simulink model "sldemo2_househeat"  (R2020b)
settings: Solver=ode45  StartTime=0.0  StopTime=48  FixedStep=1  RelTol=1e-3  AbsTol=1e-6
model workspace (MATLAB code in the model file):
  | % load initial conditions and physical properties from file
  | 
  | sldemo_househeat_data
values from neighbouring files (symbols this model uses):
  c = 1005.4    [sldemo_househeat_data.m]
  cost = 0.09/3.6e6    (= 2.5e-08)    [sldemo_househeat_data.m]
  M = (lenHouse*widHouse*htHouse+tan(pitRoof)*widHouse*lenHouse)*densAir    [sldemo_househeat_data.m]
  Mdot = 3600    [sldemo_househeat_data.m]
  Req = RWall*RWindow/(RWall + RWindow)    [sldemo_househeat_data.m]
  TCooler = 5    [sldemo_househeat_data.m]
  THeater = 50    [sldemo_househeat_data.m]
  TinIC = 20    [sldemo_househeat_data.m]
libraries: simulink_extras x3
Description:
  | Thermal Model of a House
  | 
  | This demo illustrates how you can use Simulink(R) to create the thermal model of
  | a house. This system models the outdoor environment, the thermal
  | characteristics of the house, and the house heating system.
  | 
  | The sldemo_househeat_data.m file initializes data in the model workspace.
  | To make changes, you can edit the model workspace directly or edit the MATLAB(R) file
  | and re-load the model workspace.
  | 
  | To view the model workspace, select View > Model Explorer
  | from the Simulink editor.
  | 
  | Note: Time is given in units of hours
settings Model: ExtModeTrigMode=oneshot  ExtModeArmWhenConnect=off  ExtModeAutoUpdateStatusClock=off  Creator=The MathWorks, Inc.  LastModifiedBy=91998
settings SolverCC: AutoScaleAbsTol=off
settings DataIOCC: ExternalInput=[]  InitialState=[]  SaveFormat=Array  SaveOutput=off  SaveTime=off  SignalLoggingName=sldemo_househeat_output
settings OptimizationCC: BlockReduction=off  BooleanDataType=off  ExpressionDepthLimit=2147483647  InitFltsAndDblsToZero=on  LifeSpan=inf  BufferReusableBoundary=off
settings DebuggingCC: SaveWithParameterizedLinksMsg=none  UnderspecifiedInitializationDetection=Classic  MergeDetectMultiDrivingBlocksExec=none  SignalResolutionControl=TryResolveAllWithWarning  MultiTaskDSMMsg=warning  MultiTaskCondExecSysMsg=none  IntegerOverflowMsg=none  FcnCallInpInsideContextMsg=warning  BusObjectLabelMismatch=none  StateNameClashWarn=warning  SFUnexpectedBacktrackingDiag=warning  SFNoUnconditionalDefaultTransitionDiag=warning  SFExecutionAtInitializationDiag=none  IntegerSaturationMsg=none  ArithmeticOperatorsInVariantConditions=warning
settings HardwareCC: ProdBitPerPointer=32  ProdBitPerSizeT=32  ProdBitPerPtrDiffT=32  ProdLargestAtomicFloat=None  ProdIntDivRoundTo=Undefined  ProdEndianess=Unspecified  ProdWordSize=32  ProdHWDeviceType=32-bit Generic  TargetUnknown=on
settings ModelReferenceCC: PropagateSignalLabelsOutOfModel=off
settings SFSimCC: SimUseLocalCustomCode=off  CustomCodeUndefinedFunction=UseInterfaceOnly
settings RTWCC: RTWUseLocalCustomCode=off
settings CodeAppCC: StateflowObjectComments=on
settings GRTTargetCC: TargetFcnLib=ansi_tfl_tmw.mat  TargetLangStandard=C89/C90 (ANSI)  CombineOutputUpdateFcns=off  GRTInterface=on
settings ConfigComp: CovMetricSettings=dw  CovSaveCumulativeToWorkspaceVar=on  CovSaveSingleToWorkspaceVar=on  CovExternalEMLEnable=off

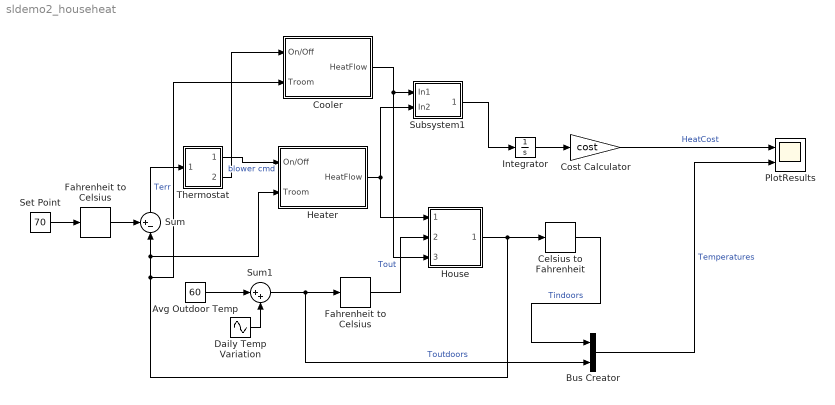
== system sldemo2_househeat ==
  Avg Outdoor Temp : Constant  Value=60
  Bus Creator : BusCreator  Inputs=3
  Celsius to Fahrenheit : simulink_extras/Transformations/Celsius to Fahrenheit
      settings: SourceProductBaseCode=SL
  Cooler : Subsystem
  Cost Calculator : Gain  Gain=cost  SaturateOnIntegerOverflow=on  OutDataTypeStr=Inherit: Same as input  ParamDataTypeStr=Inherit: Same as input
  Daily Temp Variation : Sin  Amplitude=30  Frequency=2*pi/24  SampleTime=0
  Fahrenheit to Celsius : simulink_extras/Transformations/Fahrenheit to Celsius
      settings: SourceProductBaseCode=SL
  "Fahrenheit to Celsius " : simulink_extras/Transformations/Fahrenheit to Celsius
      settings: SourceProductBaseCode=SL
  Heater : Subsystem
  House : Subsystem
      mask Display: image(fullfile(matlabroot,'toolbox','simulink','simdemos','simgeneral','images','HouseHeatHousePix.svg'))
  Integrator : Integrator
  PlotResults : Scope  NumInputPorts=2
  Set Point : Constant  Value=70
  Subsystem1 : Subsystem
  Sum : Sum  Inputs=+-|  InputSameDT=on  SaturateOnIntegerOverflow=on  OutDataTypeStr=Inherit: Same as first input
  Sum1 : Sum  Inputs=|++  InputSameDT=on  SaturateOnIntegerOverflow=on  OutDataTypeStr=Inherit: Same as first input
  Thermostat : Subsystem
      mask Display: image(fullfile(matlabroot,'toolbox','simulink','simdemos','simgeneral','images','HouseHeatThermostatPix.svg'))
  wires:
  Integrator/1 -> Cost Calculator/1
  Thermostat/1(Heater Blower switch) -> Heater/1(On/Off)  "blower cmd"
  Sum/1 -> Thermostat/1(Terr)  "Terr"
  House/1(Room Temp Troom) -> Cooler/2(Troom), Heater/2(Troom), Sum/2, Celsius to Fahrenheit/1
  Daily Temp Variation/1 -> Sum1/2
  Sum1/1 -> Fahrenheit to Celsius/1, Bus Creator/3  "Toutdoors"
  Avg Outdoor Temp/1 -> Sum1/1
  Celsius to Fahrenheit/1 -> Bus Creator/1  "Tindoors"
  Fahrenheit to Celsius/1 -> House/2(Outdoor Temp Tout)  "Tout"
  Heater/1(HeatFlow) -> House/1(Heater QDot In), Subsystem1/2(In2)
  Bus Creator/1 -> PlotResults/2  "Temperatures"
  Cost Calculator/1 -> PlotResults/1  "HeatCost"
  "Fahrenheit to Celsius "/1 -> Sum/1
  Set Point/1 -> "Fahrenheit to Celsius "/1
  Thermostat/2(Cooler Subsystem) -> Cooler/1(On/Off)
  Cooler/1(HeatFlow) -> House/3(Cooler QDot In), Subsystem1/1(In1)
  Subsystem1/1(Out1) -> Integrator/1

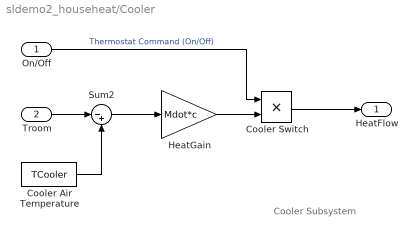
== system sldemo2_househeat/Cooler ==
  note: Cooler Subsystem
  On/Off : Inport
  Troom : Inport  Port=2
  Cooler Air Temperature : Constant  Value=TCooler
  Cooler Switch : Product  RndMeth=Zero
  HeatGain : Gain  Gain=Mdot*c
  Sum2 : Sum  Inputs=|-+
  HeatFlow : Outport  VectorParamsAs1DForOutWhenUnconnected=off
  wires:
  On/Off/1 -> Cooler Switch/1  "Thermostat Command (On/Off)"
  HeatGain/1 -> Cooler Switch/2
  Cooler Switch/1 -> HeatFlow/1
  Troom/1 -> Sum2/1
  Cooler Air Temperature/1 -> Sum2/2
  Sum2/1 -> HeatGain/1

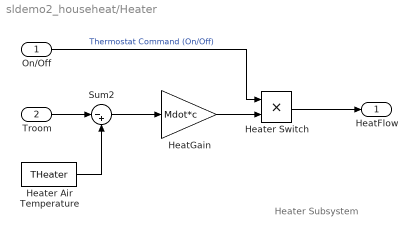
== system sldemo2_househeat/Heater ==
  note: Heater Subsystem
  On/Off : Inport
  Troom : Inport  Port=2
  HeatGain : Gain  Gain=Mdot*c
  Heater Air Temperature : Constant  Value=THeater
  Heater Switch : Product  RndMeth=Zero
  Sum2 : Sum  Inputs=|-+
  HeatFlow : Outport  VectorParamsAs1DForOutWhenUnconnected=off
  wires:
  Heater Air Temperature/1 -> Sum2/2
  Troom/1 -> Sum2/1
  Sum2/1 -> HeatGain/1
  On/Off/1 -> Heater Switch/1  "Thermostat Command (On/Off)"
  HeatGain/1 -> Heater Switch/2
  Heater Switch/1 -> HeatFlow/1

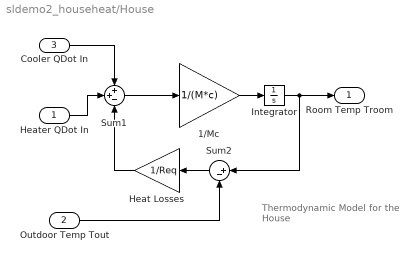
== system sldemo2_househeat/House ==
  note: Thermodynamic Model
      | for the House
  Heater QDot In : Inport
  Outdoor Temp Tout : Inport  Port=2
  Cooler QDot In : Inport  Port=3
  1/Mc : Gain  Gain=1/(M*c)  SaturateOnIntegerOverflow=on  OutDataTypeStr=Inherit: Same as input  ParamDataTypeStr=Inherit: Same as input
  Heat Losses : Gain  Gain=1/Req  SaturateOnIntegerOverflow=on  OutDataTypeStr=Inherit: Same as input  ParamDataTypeStr=Inherit: Same as input
  Integrator : Integrator  InitialCondition=TinIC
  Sum1 : Sum  Inputs=++-  InputSameDT=on  SaturateOnIntegerOverflow=on  OutDataTypeStr=Inherit: Same as first input
  Sum2 : Sum  Inputs=|+-  InputSameDT=on  SaturateOnIntegerOverflow=on  OutDataTypeStr=Inherit: Same as first input
  Room Temp Troom : Outport  InitialOutput=0  VectorParamsAs1DForOutWhenUnconnected=off
  wires:
  Outdoor Temp Tout/1 -> Sum2/2
  Sum1/1 -> 1/Mc/1
  Sum2/1 -> Heat Losses/1
  1/Mc/1 -> Integrator/1
  Integrator/1 -> Sum2/1, Room Temp Troom/1
  Heat Losses/1 -> Sum1/3
  Heater QDot In/1 -> Sum1/2
  Cooler QDot In/1 -> Sum1/1

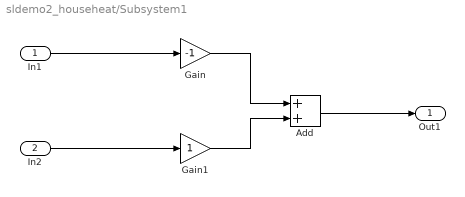
== system sldemo2_househeat/Subsystem1 ==
  In1 : Inport
  In2 : Inport  Port=2
  Add : Sum
  Gain : Gain  Gain=-1
  Gain1 : Gain
  Out1 : Outport
  wires:
  In1/1 -> Gain/1
  In2/1 -> Gain1/1
  Gain/1 -> Add/1
  Gain1/1 -> Add/2
  Add/1 -> Out1/1

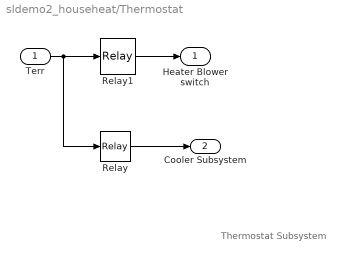
== system sldemo2_househeat/Thermostat ==
  note: Thermostat Subsystem
  Terr : Inport
  Relay : Relay  OnSwitchValue=0  OffSwitchValue=-5*(5/9)  OnOutputValue=0  OffOutputValue=1
  Relay1 : Relay  OnSwitchValue=5*(5/9)  OffSwitchValue=0
  Heater Blower switch : Outport  InitialOutput=0  VectorParamsAs1DForOutWhenUnconnected=off
  Cooler Subsystem : Outport  Port=2
  wires:
  Relay1/1 -> Heater Blower switch/1
  Terr/1 -> Relay/1, Relay1/1
  Relay/1 -> Cooler Subsystem/1
